simulink model "testTFT"  (R2017b)
settings: Solver=FixedStepDiscrete  StartTime=0.0  StopTime=40  FixedStep=1/200  RelTol=1e-3  EnableMultiTasking=on
libraries: simulink x3
settings Model: ExtModeTrigDuration=2  Creator=ndoreraj  LastModifiedBy=mgovinda
settings OptimizationCC: PassReuseOutputArgsAs=Individual arguments  MaxStackSize=64
settings DebuggingCC: ParameterTunabilityLossMsg=error
settings HardwareCC: ProdBitPerInt=16  ProdBitPerPointer=16  ProdBitPerSizeT=16  ProdBitPerPtrDiffT=16  ProdLargestAtomicFloat=None  ProdWordSize=8  ProdHWDeviceType=Atmel->AVR
settings SFSimCC: MATLABDynamicMemAlloc=off
settings RTWCC: SystemTargetFile=ert.tlc  HardwareBoard=Arduino Uno  TLCOptions=-aInlineSetEventsForThisBaseRateFcn=TLC_FALSE -aSuppressMultiTaskScheduler=TLC_FALSE -aRateBasedStepFcn=1  TemplateMakefile=ert_default_tmf  GenerateReport=on  Toolchain=Arduino AVR  BuildConfiguration=Faster Runs  IncludeHyperlinkInReport=on  LaunchReport=on  GenerateTraceInfo=on  GenerateTraceReport=on  GenerateTraceReportSl=on  GenerateTraceReportSf=on  GenerateTraceReportEml=on
settings CodeAppCC: ForceParamTrailComments=on  IgnoreCustomStorageClasses=off  OperatorAnnotations=on  SimulinkDataObjDesc=on  SFDataObjDesc=on  InsertBlockDesc=on
settings ERTTargetCC: SupportContinuousTime=on  SupportVariableSizeSignals=on

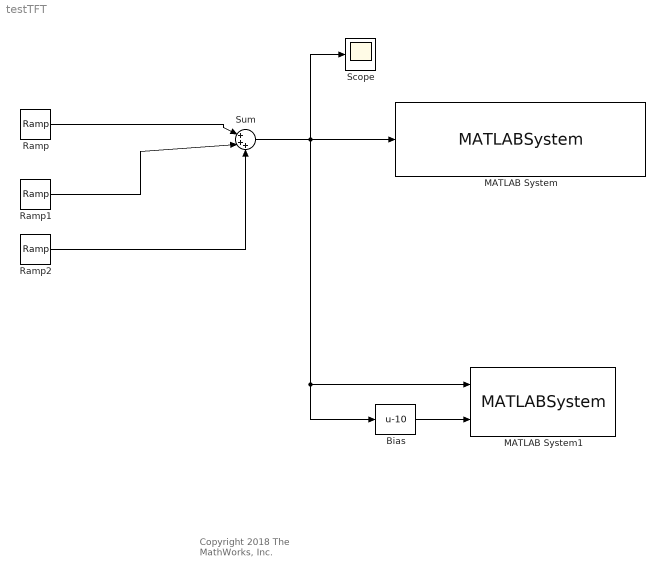
== system testTFT ==
  note: Copyright 2018 The MathWorks, Inc.
  Bias : Bias  Bias=-10
  MATLAB System : MATLABSystem  System=displayHR  txtColor_=Yellow  txtSize_=uint8( 5 )  x_=0  y_=0
      mask Type: displayHR
      mask Display:
      | disp('Display Heart Rate');
      | port_label('input',1,'Heart Rate');
  MATLAB System1 : MATLABSystem  System=displaySig  line1Color_=Green  line2Color_=Red
      mask Type: displaySig
      mask Display:
      | disp('ECG Signal Display');
      | port_label('input',1,'Raw Data');
      | port_label('input',2,'Filtered Data');
  Ramp : simulink/Sources/Ramp  slope=10  start=1  X0=0
  Ramp1 : simulink/Sources/Ramp  slope=-20  start=15  X0=0
  Ramp2 : simulink/Sources/Ramp  slope=10  start=29  X0=0
  Scope : Scope
  Sum : Sum  Inputs=|+++
  wires:
  Sum/1 -> MATLAB System/1, Bias/1, MATLAB System1/1, Scope/1
  Ramp/1 -> Sum/1
  Ramp1/1 -> Sum/2
  Ramp2/1 -> Sum/3
  Bias/1 -> MATLAB System1/2
